simulink library "BandSplitLibDeprecated"  (R2022b)
settings: Solver=VariableStepAuto  StartTime=0.0  StopTime=10.0  RelTol=1e-3
libraries: FirEven x1, HandyTextFile x1, Ifir x1, dspmlti4 x1
settings Model: Creator=jb1046154  LastModifiedBy=sa1045272
settings SolverCC: AlgebraicLoopSolver=TrustRegion
settings DebuggingCC: UnconnectedInputMsg=warning  UnconnectedOutputMsg=warning  UnconnectedLineMsg=warning  SFMachineParentedDataDiag=warning
settings ModelReferenceCC: EnableRefExpFcnMdlSchedulingChecks=on

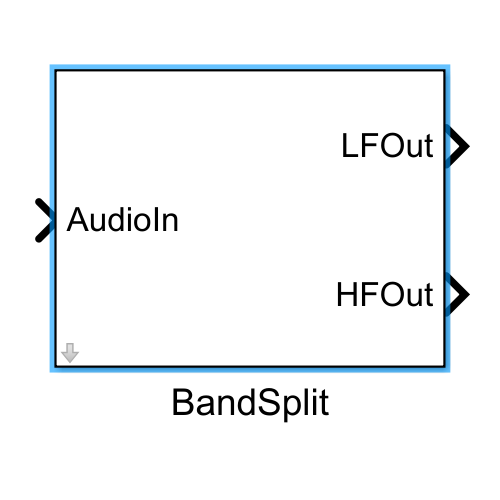
[thumbnail: Simulink's stored preview of the top-level diagram]
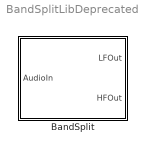
== system BandSplitLibDeprecated ==
  BandSplit : Subsystem  mask(NEAR BandSplit){Config=[]}
      mask prompts: Config "BandSplitConfig"
      mask help:
      | This mask allows the setting of parameters for version 1.1 of the NEAR BandSplit model.
      | Model parameters are set by a class instance in the base workspace.
      |
      | See 'Help' for details.
      mask init:
      | blkh=gcbh;
      | Config=BTConfig.Assert(blkh,Config);
      | 
      | Config.Validate();
      | Config.DoMaskInit(blkh);
      mask Help:
      | Defining model parameters:
      | The model parameters are set by the conents of an instance of BandSplitConfig.m.
      | 
      | To set model parameters:
      | 1-Create an instance of BandSplitConfig.m in the base workspace.
      | 2-In the model mask, set the 'Class instance' parameter to the name of the class instance in the base workspace.

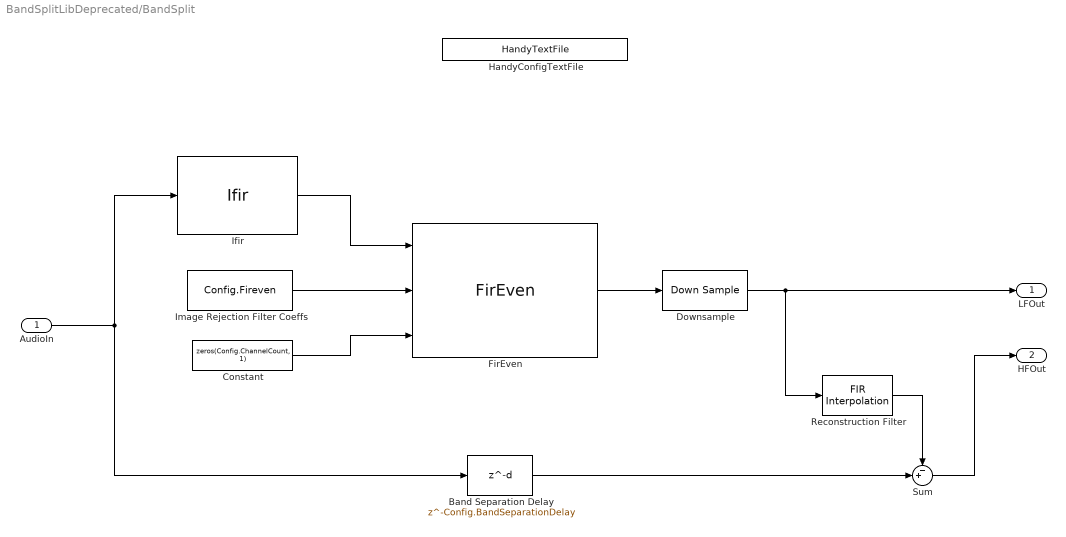
== system BandSplitLibDeprecated/BandSplit ==
  AudioIn : Inport
  Band Separation Delay : Delay  DelayLength=Config.BandSeparationDelay  InputProcessing=Columns as channels (frame based)
  Constant : Constant  Value=zeros(Config.ChannelCount, 1)  OutDataTypeStr=uint32
  Downsample : DownSample  N=Config.DecimationFactor
  FirEven : FirEven/FirEven  Config=Config.FirEven
      settings: SourceProductName=Bose Blocklib
  HandyConfigTextFile : HandyTextFile/HandyTextFile  TemplateSource=Config  FileSuffix=File  OpenDialogOnLoad=off  UseThisBlockName=off  AddGrandParentNamePrefix=off  TheDefaultText=% $(FILENAME) $(PREFIX) $(SUFFIX)  ShowInLibBrowser=on
      settings: SourceProductName=Bose Talaria
  Ifir : Ifir/Ifir  Config=Config.Ifir
  Image Rejection Filter Coeffs : Constant  Value=Config.Fireven
  Reconstruction Filter : dspmlti4/FIR Interpolation  FilterSource=Dialog parameters  PrivateCoeffs=0  h=Config.Upfir  L=Config.DecimationFactor  FilterObject=FINTERP  InputProcessing=Columns as channels (frame based)  framing=Enforce single-rate processing  outputBufInitCond=0  roundingMode=Floor  overflowMode=off  firstCoeffDataTypeStr=Inherit: Same word length as input  firstCoeffMin=[]  firstCoeffMax=[]  firstCoeffLastDataTypeStr=Inherit: Same word length as input  outputDataTypeStr=Inherit: Same as accumulator  outputMin=[]  outputMax=[]  outputLastDataTypeStr=Inherit: Same as accumulator
  Sum : Sum  Inputs=-+|
  LFOut : Outport  VectorParamsAs1DForOutWhenUnconnected=off
  HFOut : Outport  Port=2  VectorParamsAs1DForOutWhenUnconnected=off
  wires:
  Sum/1 -> HFOut/1
  Downsample/1 -> LFOut/1, Reconstruction Filter/1
  Reconstruction Filter/1 -> Sum/1
  Band Separation Delay/1 -> Sum/2
  Constant/1 -> FirEven/3
  Ifir/1 -> FirEven/1
  Image Rejection Filter Coeffs/1 -> FirEven/2
  AudioIn/1 -> Ifir/1, Band Separation Delay/1
  FirEven/1 -> Downsample/1
